simulink model "Cycloconverter"  (R2023b)
settings: Solver=VariableStepDiscrete  StartTime=0.0  StopTime=0.1  RelTol=1e-3
libraries: spsThyristorLib x8, spsIdealSwitchLib x4, spsVoltageMeasurementLib x2, spsACVoltageSourceLib x1, spsSeriesRLCBranchLib x1, sps_lib x1
settings Model: Creator=HP  LastModifiedBy=HP

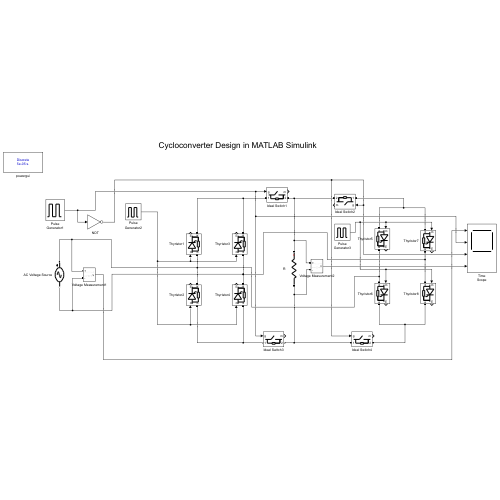
[thumbnail: Simulink's stored preview of the top-level diagram]
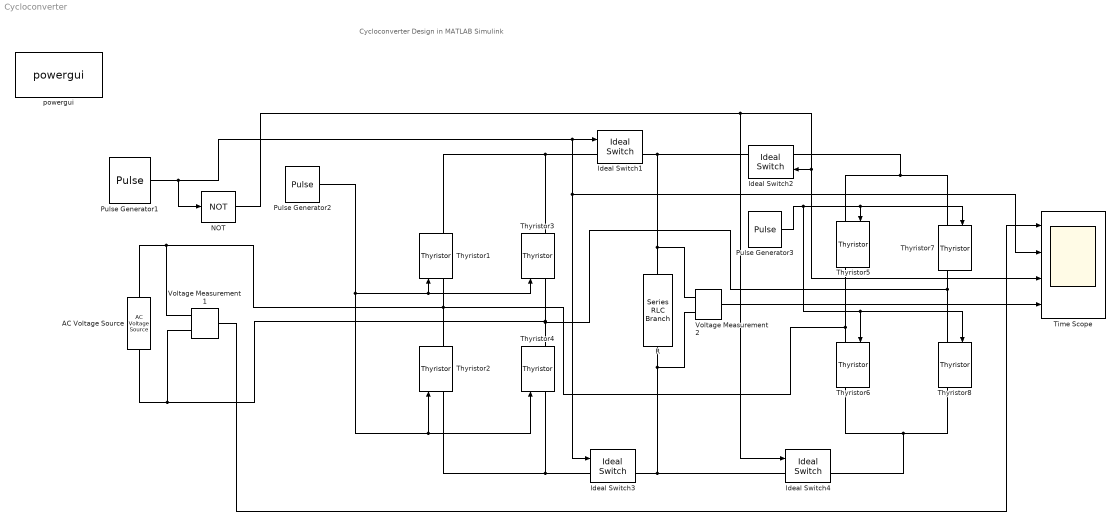
== system Cycloconverter ==
  note: Cycloconverter Design in MATLAB Simulink
  AC Voltage Source : spsACVoltageSourceLib/AC Voltage Source  Amplitude=230  Phase=0  Frequency=50  SampleTime=0  Measurements=None  BusType=swing  Pref=10e3  Qref=0  Qmin=-inf  Qmax=+inf
  Ideal Switch{1..4} (4 alike) : spsIdealSwitchLib/Ideal Switch  Ron=0.001  Lon=0  IC=0  Rs=1e5  Cs=inf  Measurements=on
  NOT : Logic  Operator=NOT  IconShape=distinctive  AllPortsSameDT=off  OutDataTypeStr=boolean
  Pulse Generator1 : DiscretePulseGenerator  PulseType=Time based  Period=0.08  PulseWidth=50
  Pulse Generator2 : DiscretePulseGenerator  PulseType=Time based  Period=0.01  PulseWidth=5  PhaseDelay=0.004
  Pulse Generator3 : DiscretePulseGenerator  PulseType=Time based  Period=0.01  PulseWidth=5  PhaseDelay=0.004
  R : spsSeriesRLCBranchLib/Series RLC Branch  LConnTagsString=__new0  RConnTagsString=__new0  BranchType=R  Resistance=1  Inductance=1e-3  SetiL0=off  InitialCurrent=0  Capacitance=1e-6  Setx0=off  InitialVoltage=0  Measurements=None
  Thyristor{1..8} (8 alike) : spsThyristorLib/Thyristor  Ron=0.001  Lon=0  Vf=0.8  IC=0  Rs=500  Cs=250e-9  Measurements=on
  Time Scope : Scope  NumInputPorts=4
  Voltage Measurement1 : spsVoltageMeasurementLib/Voltage Measurement  PhasorSimulation=off  OutputType=Complex  PSBequivalent=0
  Voltage Measurement2 : spsVoltageMeasurementLib/Voltage Measurement  PhasorSimulation=off  OutputType=Complex  PSBequivalent=0
  powergui : sps_lib/powergui  Priority=1  SimulationMode=Discrete  SampleTime=50e-6  frequency=60  Iterations=50  frequencyindice=50  Pbase=100e6  ErrMax=1e-4  UnitsV=kV  UnitsW=MW  buscounter=0  FunctionMessages=off  echomessages=off  EnableUseOfTLC=off  CurrentSourceSwitches=off  DisableSnubberDevices=off  DisableRonSwitches=off  DisableVfSwitches=off  DisplayEquations=off  AutomaticDiscreteSolvers=off  SolverType=Tustin/Backward Euler (TBE)  Interpol=off  ExternalGateDelay=off  methode=off  Ts=100  x0status=blocks  SPID=on  SwTol=0  HookPort=off  NonlinearTolerance=1e-4  nMaxIteration=100  ContinueOnMaxIteration=off  RestoreLinks=warning  ResistiveCurrentMeasurement=off  Frange=[0:2:500]  Ylog=off  Xlog=on  ShowGrid=off  save=off  variable=ZData  structure=0  ZoomFFT=off  StartTime=0.0  cycles=1  DisplayStyle=1  fundamental=60  FreqAxis=off  MaxFrequency=1000  frequencyindicesteady=1  RmsSteady=1  display=off
  wires:
  Pulse Generator2/1 -> Thyristor3/1, Thyristor1/1, Thyristor2/1, Thyristor4/1
  Pulse Generator1/1 -> NOT/1, Ideal Switch3/1, Time Scope/2, Ideal Switch1/1
  NOT/1 -> Time Scope/3, Ideal Switch2/1, Ideal Switch4/1
  Pulse Generator3/1 -> Thyristor8/1, Thyristor6/1, Thyristor7/1, Thyristor5/1
  Voltage Measurement1/1 -> Time Scope/1
  Voltage Measurement2/1 -> Time Scope/4
  connections:
  Thyristor4/RConn1 -- Thyristor8/LConn1 -- Thyristor7/RConn1 -- Voltage Measurement1/LConn2 -- AC Voltage Source/LConn1 -- Thyristor3/LConn1
  Thyristor1/RConn1 -- Thyristor3/RConn1 -- Ideal Switch1/LConn1
  Thyristor2/LConn1 -- Thyristor4/LConn1 -- Ideal Switch3/LConn1
  Thyristor1/LConn1 -- Thyristor5/RConn1 -- Thyristor6/LConn1 -- Thyristor2/RConn1 -- Voltage Measurement1/LConn1 -- AC Voltage Source/RConn1
  Ideal Switch1/RConn1 -- Ideal Switch2/RConn1 -- R/LConn1 -- Voltage Measurement2/LConn1
  Ideal Switch3/RConn1 -- Ideal Switch4/LConn1 -- R/RConn1 -- Voltage Measurement2/LConn2
  Thyristor5/LConn1 -- Ideal Switch2/LConn1 -- Thyristor7/LConn1
  Thyristor6/RConn1 -- Ideal Switch4/RConn1 -- Thyristor8/RConn1
